simulink model "EvitaParedes_US_016"  (R2023b)
settings: Solver=VariableStepAuto  StartTime=0.0  StopTime=10.0  RelTol=1e-3
settings Model: Creator=Usuario_UMA  LastModifiedBy=javie

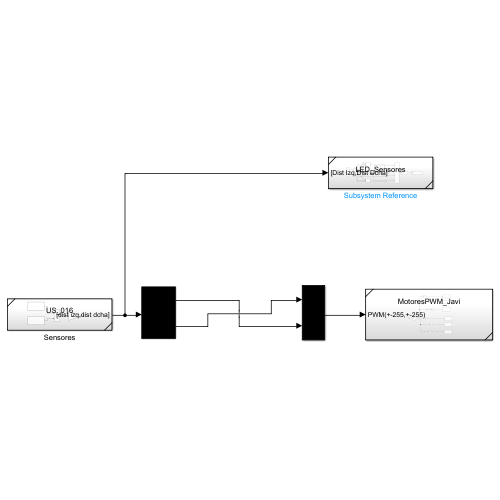
[thumbnail: Simulink's stored preview of the top-level diagram]
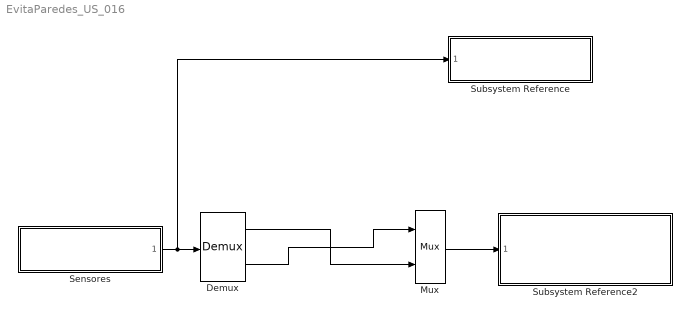
== system EvitaParedes_US_016 ==
  Demux : Demux  Outputs=2
  Mux : Mux  Inputs=2
  Sensores : Subsystem  ReferencedSubsystem=US_016
  Subsystem Reference : Subsystem  ReferencedSubsystem=LED_Sensores
  Subsystem Reference2 : Subsystem  ReferencedSubsystem=MotoresPWM_Javi
  wires:
  Mux/1 -> Subsystem Reference2/1
  Sensores/1 -> Subsystem Reference/1, Demux/1
  Demux/1 -> Mux/2
  Demux/2 -> Mux/1
